simulink model "Speed_Control"  (R2017a)
settings: Solver=VariableStepAuto  StartTime=0.0  StopTime=tmax  RelTol=1e-3
values from neighbouring files (symbols this model uses):
  B = 0.1    [No2.mat]    (also in simTest.m = [b 0 ; 0 beta])
  J = 2    [No2.mat]
  Kb = 1    [No2.mat]
  Ki = 70    [No2.mat]
  Km = 10    [No2.mat]
  Kp = 150    [No2.mat]
  L = 0.1    [No2.mat]
  r = 20    [No2.mat]
  R = 10    [No2.mat]
libraries: simulink x2
settings Model: Creator=USER  LastModifiedBy=Sorawit Inprom

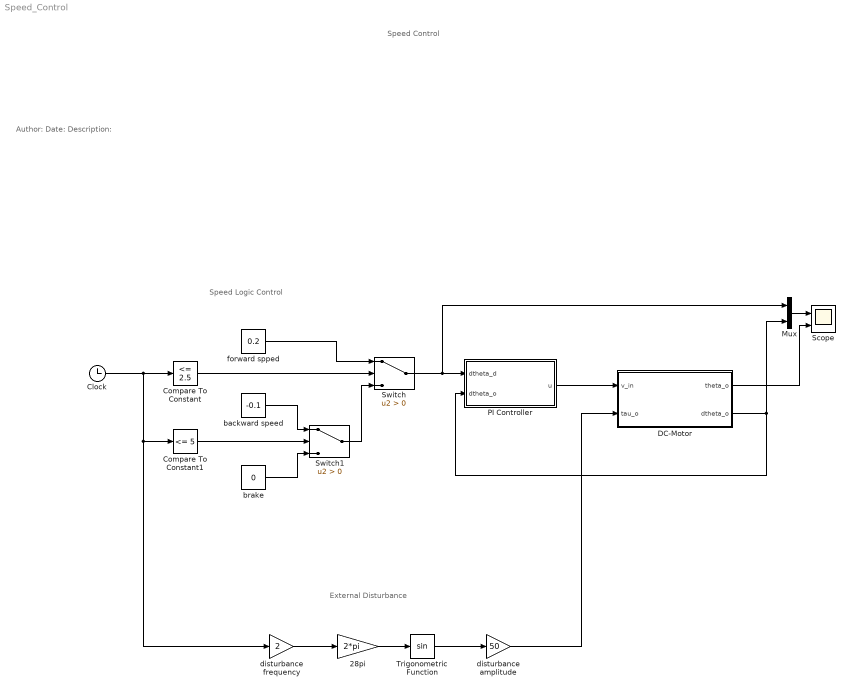
== system Speed_Control ==
  note: Speed Control
  note: Author:
      | Date:
      | Description:
  note: External Disturbance
  note: Speed Logic Control
  28pi : Gain  Gain=2*pi
  Clock : Clock
  Compare To Constant : simulink/Logic and Bit Operations/Compare To Constant  relop=<=  const=2.5  OutDataTypeStr=boolean
  Compare To Constant1 : simulink/Logic and Bit Operations/Compare To Constant  relop=<=  const=5  OutDataTypeStr=boolean
  DC-Motor : Subsystem
  Mux : Mux  Inputs=2
  PI Controller : Subsystem
  Scope : Scope  NumInputPorts=2
  Switch : Switch  Criteria=u2 > Threshold
  Switch1 : Switch  Criteria=u2 > Threshold
  Trigonometric Function : Trigonometry
  backward speed : Constant  Value=-0.1
  brake : Constant  Value=0
  disturbance amplitude : Gain  Gain=50
  disturbance frequency : Gain  Gain=2
  forward spped : Constant  Value=0.2
  wires:
  PI Controller/1(u) -> DC-Motor/1(v_in)
  Switch1/1 -> Switch/3
  forward spped/1 -> Switch/1
  backward speed/1 -> Switch1/1
  brake/1 -> Switch1/3
  Compare To Constant/1 -> Switch/2
  Compare To Constant1/1 -> Switch1/2
  Clock/1 -> Compare To Constant/1, Compare To Constant1/1, disturbance frequency/1
  disturbance frequency/1 -> 28pi/1
  28pi/1 -> Trigonometric Function/1
  Trigonometric Function/1 -> disturbance amplitude/1
  disturbance amplitude/1 -> DC-Motor/2(tau_o)
  Switch/1 -> Mux/1, PI Controller/1(dtheta_d)
  DC-Motor/2(dtheta_o) -> PI Controller/2(dtheta_o), Mux/2
  Mux/1 -> Scope/1
  DC-Motor/1(theta_o) -> Scope/2

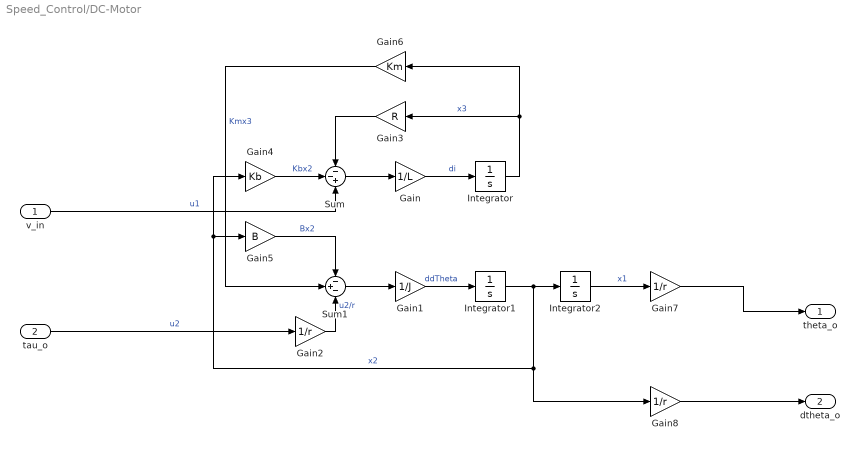
== system Speed_Control/DC-Motor ==
  v_in : Inport
  tau_o : Inport  Port=2
  Gain : Gain  Gain=1/L
  Gain1 : Gain  Gain=1/J
  Gain2 : Gain  Gain=1/r
  Gain3 : Gain  Gain=R
  Gain4 : Gain  Gain=Kb
  Gain5 : Gain  Gain=B
  Gain6 : Gain  Gain=Km
  Gain7 : Gain  Gain=1/r
  Gain8 : Gain  Gain=1/r
  Integrator : Integrator
  Integrator1 : Integrator
  Integrator2 : Integrator
  Sum : Sum  Inputs=--+
  Sum1 : Sum  Inputs=-+-
  theta_o : Outport
  dtheta_o : Outport  Port=2
  wires:
  Gain/1 -> Integrator/1  "di"
  Integrator/1 -> Gain6/1, Gain3/1  "x3"
  Integrator1/1 -> Gain8/1, Gain4/1, Gain5/1, Integrator2/1  "x2"
  Gain1/1 -> Integrator1/1  "ddTheta"
  Integrator2/1 -> Gain7/1  "x1"
  Sum/1 -> Gain/1
  tau_o/1 -> Gain2/1  "u2"
  v_in/1 -> Sum/3  "u1"
  Gain3/1 -> Sum/1
  Gain4/1 -> Sum/2  "Kbx2"
  Gain5/1 -> Sum1/1  "Bx2"
  Gain2/1 -> Sum1/3  "u2/r"
  Sum1/1 -> Gain1/1
  Gain7/1 -> theta_o/1
  Gain8/1 -> dtheta_o/1
  Gain6/1 -> Sum1/2  "Kmx3"

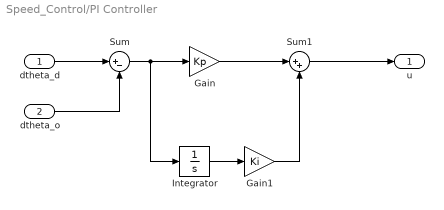
== system Speed_Control/PI Controller ==
  dtheta_d : Inport
  dtheta_o : Inport  Port=2
  Gain : Gain  Gain=Kp
  Gain1 : Gain  Gain=Ki
  Integrator : Integrator
  Sum : Sum  Inputs=|+-
  Sum1 : Sum  Inputs=|++
  u : Outport
  wires:
  dtheta_d/1 -> Sum/1
  dtheta_o/1 -> Sum/2
  Sum/1 -> Integrator/1, Gain/1
  Gain/1 -> Sum1/1
  Gain1/1 -> Sum1/2
  Integrator/1 -> Gain1/1
  Sum1/1 -> u/1
